simulink model "rigid_body_model_translation"  (R2021a)
settings: Solver=ode4  StartTime=0.0  StopTime=10.0  RelTol=1e-3
libraries: dspinverses x1, vrlib x1
settings Model: Creator=jadg1  LastModifiedBy=jadg1

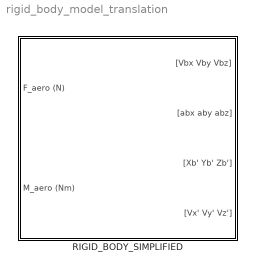
== system rigid_body_model_translation ==
  RIGID_BODY_SIMPLIFIED : Subsystem

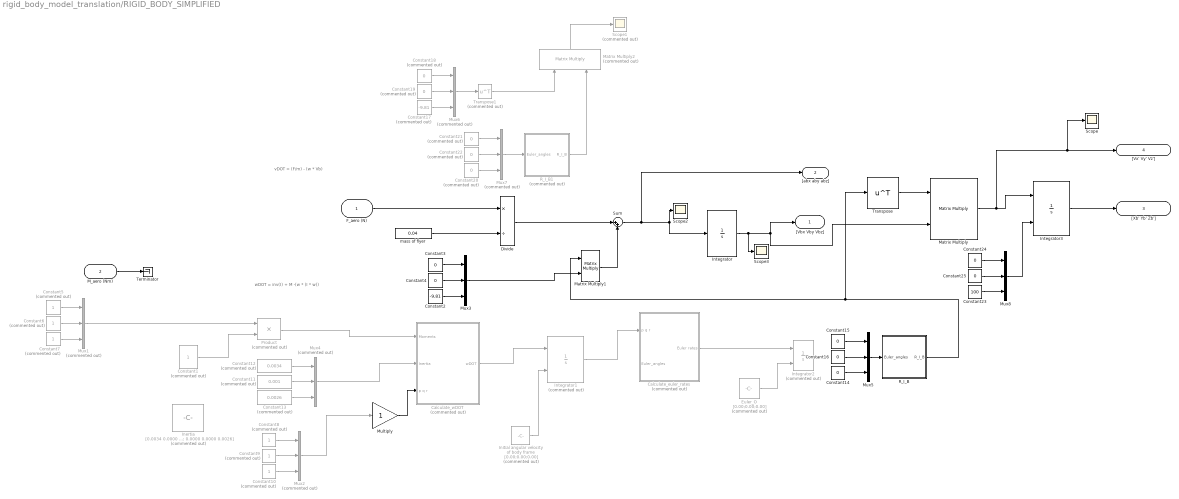
== system rigid_body_model_translation/RIGID_BODY_SIMPLIFIED ==
  note: wDOT = inv(I) + M -(w * (I * w))
  note: vDOT = (F/m) - (w * Vb)
  F_aero (N) : Inport
  M_aero (Nm) : Inport  Port=2
  Calculate_euler_rates : Subsystem  Commented=on
  Calculate_wDOT : Subsystem  Commented=on
  Constant{1,5..10} (7 alike) : Constant  Commented=on
  Constant11 : Constant  Commented=on  Value=0.001
  Constant12 : Constant  Commented=on  Value=0.0034
  Constant13 : Constant  Commented=on  Value=0.0026
  Constant{3..4,14..16,24..25} (7 alike) : Constant  Value=0
  Constant17 : Constant  Commented=on  Value=-9.81
  Constant{18..22} (5 alike) : Constant  Commented=on  Value=0
  Constant2 : Constant  Value=-9.81
  Constant23 : Constant  Value=100
  Divide : Product  Inputs=*/
  Euler_O : Constant  Commented=on  Value=[0.00;0.00;0.00]
  Inertia : Constant  Commented=on  Value=[0.0034 0.0000 0.0000; 0.0000 0.0010 0.0000; 0.0000 0.0000 0.0026]
  Initial angular velocity of body frame : Constant  Commented=on  Value=[0.00;0.00;0.00]
  Integrator : Integrator
  Integrator1 : Integrator  Commented=on  InitialConditionSource=external
  Integrator2 : Integrator  Commented=on  InitialConditionSource=external
  Integrator3 : Integrator  InitialConditionSource=external
  Matrix Multiply : Product  Multiplication=Matrix(*)
  Matrix Multiply1 : Product  Multiplication=Matrix(*)
  Matrix Multiply2 : Product  Commented=on  Multiplication=Matrix(*)
  Multiply : Gain
  Mux{1..2,4,6..7} (5 alike) : Mux  Commented=on  Inputs=3
  Mux3 : Mux  Inputs=3
  Mux5 : Mux  Inputs=3
  Mux8 : Mux  Inputs=3
  Product : Product  Commented=on
  R_I_B : Subsystem
  R_I_B1 : Subsystem  Commented=on
  Scope : Scope
  Scope1 : Scope  Commented=on
  Scope2 : Scope
  Scope3 : Scope
  Sum : Sum  Inputs=|++
  Terminator : Terminator
  Transpose : Math  Operator=transpose  SaturateOnIntegerOverflow=on
  Transpose1 : Math  Commented=on  Operator=transpose  SaturateOnIntegerOverflow=on
  mass of flyer : Constant  Value=0.04
  "[Vbx Vby Vbz]" : Outport
  "[abx aby abz]" : Outport  Port=2
  "[Xb' Yb' Zb']" : Outport  Port=3
  "[Vx' Vy' Vz']" : Outport  Port=4
  wires:
  mass of flyer/1 -> Divide/2
  M_aero (Nm)/1 -> Terminator/1
  Constant8/1 -> Mux2/1
  Euler_O/1 -> Integrator2/2
  Constant9/1 -> Mux2/2
  Product/1 -> Calculate_wDOT/1(Moments)
  F_aero (N)/1 -> Divide/1
  Constant13/1 -> Mux4/3
  Transpose/1 -> Matrix Multiply/1
  Initial angular velocity of body frame/1 -> Integrator1/2
  Integrator/1 -> Scope3/1, Matrix Multiply/2, "[Vbx Vby Vbz]"/1
  Integrator1/1 -> Calculate_euler_rates/1(p q r)
  Constant10/1 -> Mux2/3
  Mux4/1 -> Calculate_wDOT/2(Inertia)
  Constant12/1 -> Mux4/1
  Calculate_euler_rates/1(Euler rates) -> Integrator2/1
  Constant11/1 -> Mux4/2
  Mux2/1 -> Multiply/1
  Multiply/1 -> Calculate_wDOT/3(p q r)
  Matrix Multiply/1 -> "[Vx' Vy' Vz']"/1, Scope/1, Integrator3/1
  R_I_B/1(R_I_B) -> Transpose/1, Matrix Multiply1/1
  Constant1/1 -> Product/2
  Calculate_wDOT/1(wDOT) -> Integrator1/1
  Constant5/1 -> Mux1/1
  Constant6/1 -> Mux1/2
  Mux1/1 -> Product/1
  Constant7/1 -> Mux1/3
  Integrator3/1 -> "[Xb' Yb' Zb']"/1
  Constant16/1 -> Mux5/2
  Constant15/1 -> Mux5/1
  Mux5/1 -> R_I_B/1(Euler_angles)
  Constant14/1 -> Mux5/3
  Divide/1 -> Sum/1
  Sum/1 -> "[abx aby abz]"/1, Scope2/1, Integrator/1
  Constant2/1 -> Mux3/3
  Constant3/1 -> Mux3/1
  Constant4/1 -> Mux3/2
  Constant18/1 -> Mux6/1
  Constant19/1 -> Mux6/2
  Constant17/1 -> Mux6/3
  Constant20/1 -> Mux7/3
  Constant21/1 -> Mux7/1
  Constant22/1 -> Mux7/2
  Matrix Multiply2/1 -> Scope1/1
  Mux7/1 -> R_I_B1/1(Euler_angles)
  Mux6/1 -> Transpose1/1
  Transpose1/1 -> Matrix Multiply2/1
  R_I_B1/1(R_I_B) -> Matrix Multiply2/2
  Matrix Multiply1/1 -> Sum/2
  Mux3/1 -> Matrix Multiply1/2
  Mux8/1 -> Integrator3/2
  Constant23/1 -> Mux8/3
  Constant25/1 -> Mux8/2
  Constant24/1 -> Mux8/1

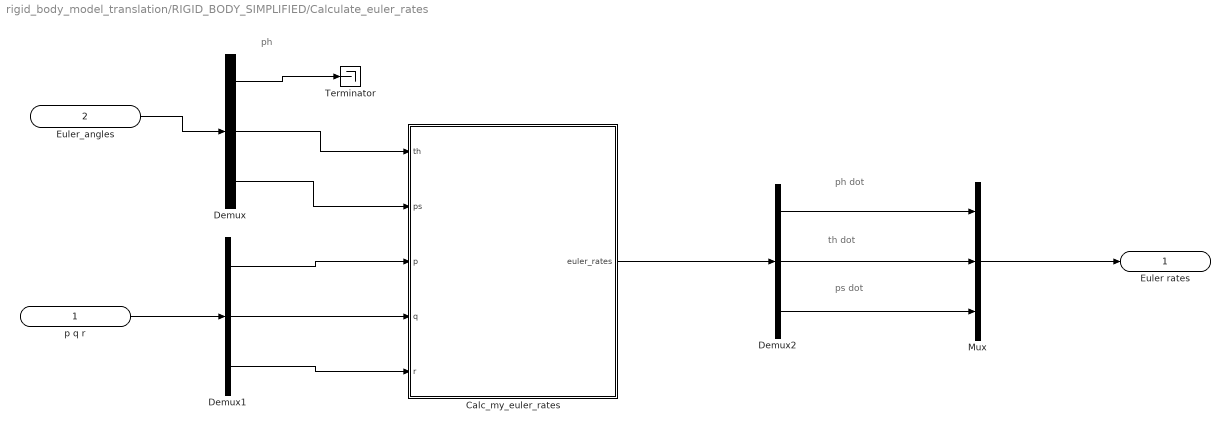
== system rigid_body_model_translation/RIGID_BODY_SIMPLIFIED/Calculate_euler_rates ==
  note: ps dot
  note: th dot
  note: ph dot
  note: ph
  p q r : Inport
  Euler_angles : Inport  Port=2
  Calc_my_euler_rates : MATLAB Function  TreatAsAtomicUnit=on
  Demux : Demux  Outputs=[-1;1;1]
  Demux1 : Demux  Outputs=[1;1;1]
  Demux2 : Demux  Outputs=3
  Mux : Mux  Inputs=3
  Terminator : Terminator
  Euler rates : Outport
  wires:
  Demux/1 -> Terminator/1
  Euler_angles/1 -> Demux/1
  Demux/2 -> Calc_my_euler_rates/1(th)
  Demux/3 -> Calc_my_euler_rates/2(ps)
  p q r/1 -> Demux1/1
  Demux1/2 -> Calc_my_euler_rates/4(q)
  Demux1/1 -> Calc_my_euler_rates/3(p)
  Demux1/3 -> Calc_my_euler_rates/5(r)
  Calc_my_euler_rates/1(euler_rates) -> Demux2/1
  Demux2/2 -> Mux/2
  Demux2/1 -> Mux/1
  Demux2/3 -> Mux/3
  Mux/1 -> Euler rates/1

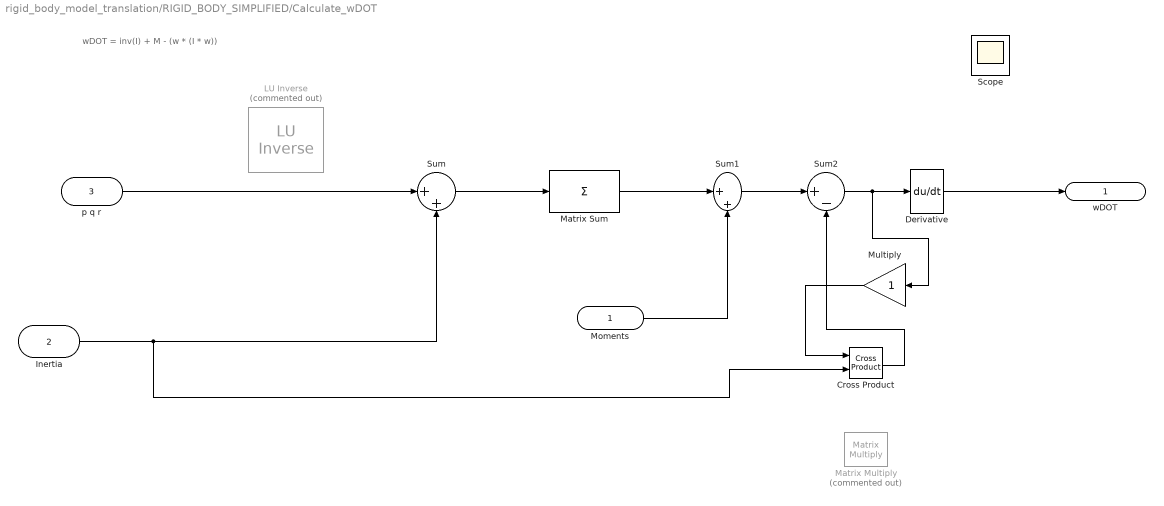
== system rigid_body_model_translation/RIGID_BODY_SIMPLIFIED/Calculate_wDOT ==
  note: wDOT = inv(I) + M - (w * (I * w))
  Moments : Inport
  Inertia : Inport  Port=2
  p q r : Inport  Port=3
  " LU Inverse" : dspinverses/ LU Inverse  Commented=on
  Cross Product : vrlib/Utilities/Cross Product
  Derivative : Derivative
  Matrix Sum : Sum  Inputs=+
  Matrix Multiply : Product  Commented=on  Multiplication=Matrix(*)
  Multiply : Gain
  Scope : Scope
  Sum : Sum  Inputs=|++
  Sum1 : Sum  Inputs=|++
  Sum2 : Sum  Inputs=|+-
  wDOT : Outport
  wires:
  Sum/1 -> Matrix Sum/1
  Matrix Sum/1 -> Sum1/1
  Sum1/1 -> Sum2/1
  Multiply/1 -> Cross Product/1
  Sum2/1 -> Multiply/1, Derivative/1
  Cross Product/1 -> Sum2/2
  Derivative/1 -> wDOT/1
  Moments/1 -> Sum1/2
  p q r/1 -> Sum/1
  Inertia/1 -> Cross Product/2, Sum/2

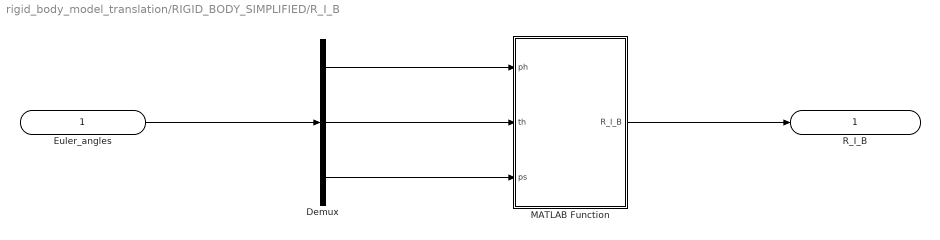
== system rigid_body_model_translation/RIGID_BODY_SIMPLIFIED/R_I_B ==
  Euler_angles : Inport
  Demux : Demux  Outputs=[1;1;1]
  MATLAB Function : MATLAB Function  TreatAsAtomicUnit=on
  R_I_B : Outport
  wires:
  Euler_angles/1 -> Demux/1
  Demux/2 -> MATLAB Function/2(th)
  Demux/3 -> MATLAB Function/3(ps)
  Demux/1 -> MATLAB Function/1(ph)
  MATLAB Function/1(R_I_B) -> R_I_B/1

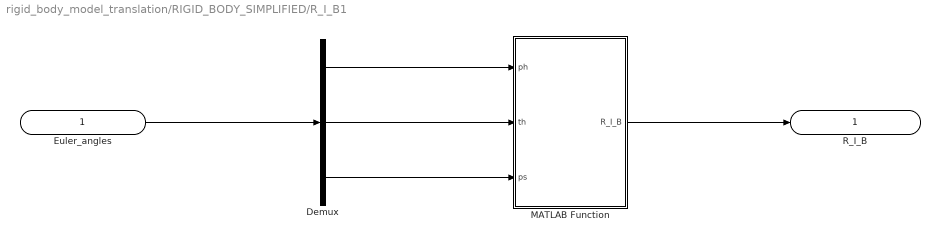
== system rigid_body_model_translation/RIGID_BODY_SIMPLIFIED/R_I_B1 ==
  Euler_angles : Inport
  Demux : Demux  Outputs=[1;1;1]
  MATLAB Function : MATLAB Function  TreatAsAtomicUnit=on
  R_I_B : Outport
  wires:
  Euler_angles/1 -> Demux/1
  Demux/2 -> MATLAB Function/2(th)
  Demux/3 -> MATLAB Function/3(ps)
  Demux/1 -> MATLAB Function/1(ph)
  MATLAB Function/1(R_I_B) -> R_I_B/1

== matlab function rigid_body_model_translation/RIGID_BODY_SIMPLIFIED/Calculate_euler_rates/Calc_my_euler_rates ==
  data: th input; euler_rates output; ps input; p input; q input; r input
function euler_rates = my_euler_rates(th,ps,p,q,r)
euler_rates = [(r .* cos(ps) + q .* sin(ps)) ./ cos(th);
                q .* cos(ps) - r .* sin(ps);
                (p .* cos(th) + r.* cos(ps) .* sin(th) + q .* sin(ps) .* sin(th)) ./ cos(th)];
end

== matlab function rigid_body_model_translation/RIGID_BODY_SIMPLIFIED/R_I_B/MATLAB Function ==
  data: ph input; R_I_B output; th input; ps input
function R_I_B = calc_R_I_B(ph, th, ps)

R_I_B = [cos(th)*cos(ps)              cos(th)*sin(ps)              -sin(th);
               sin(ph)*sin(th)*cos(ps)-cos(ph)*sin(ps)  sin(ph)*sin(th)*sin(ps)+cos(ph)*cos(ps)  sin(ph)*cos(th);
               cos(ph)*sin(th)*cos(ps)+sin(ph)*sin(ps)  cos(ph)*sin(th)*sin(ps)-sin(ph)*cos(ps)  cos(ph)*cos(th)];
end

== matlab function rigid_body_model_translation/RIGID_BODY_SIMPLIFIED/R_I_B1/MATLAB Function ==
  data: ph input; R_I_B output; th input; ps input
function R_I_B = calc_R_I_B(ph, th, ps)

R_I_B = [cos(th)*cos(ps)              cos(th)*sin(ps)              -sin(th);
               sin(ph)*sin(th)*cos(ps)-cos(ph)*sin(ps)  sin(ph)*sin(th)*sin(ps)+cos(ph)*cos(ps)  sin(ph)*cos(th);
               cos(ph)*sin(th)*cos(ps)+sin(ph)*sin(ps)  cos(ph)*sin(th)*sin(ps)-sin(ph)*cos(ps)  cos(ph)*cos(th)];
end
